simulink model "ASSIGN_pe_q12"  (R2025b)
settings: Solver=VariableStepAuto  StartTime=0.0  StopTime=0.5  RelTol=1e-3
libraries: spsACVoltageSourceLib x3, spsThyristorLib x3, spsGroundLib x2, spsRMSLib x2, spsVoltageMeasurementLib x2, spsCurrentMeasurementLib x1, spsMeanLib x1, spsPower3phInstantaneousLib x1, spsSeriesRLCBranchLib x1, spsThreePhaseVIMeasurementLib x1, sps_lib x1
settings Model: Creator=Luqmaan  LastModifiedBy=Luqmaan

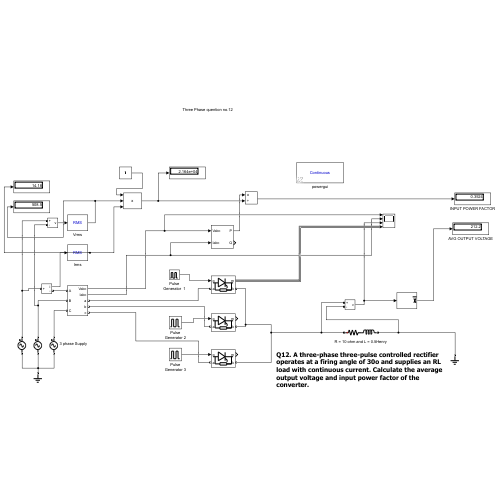
[thumbnail: Simulink's stored preview of the top-level diagram]
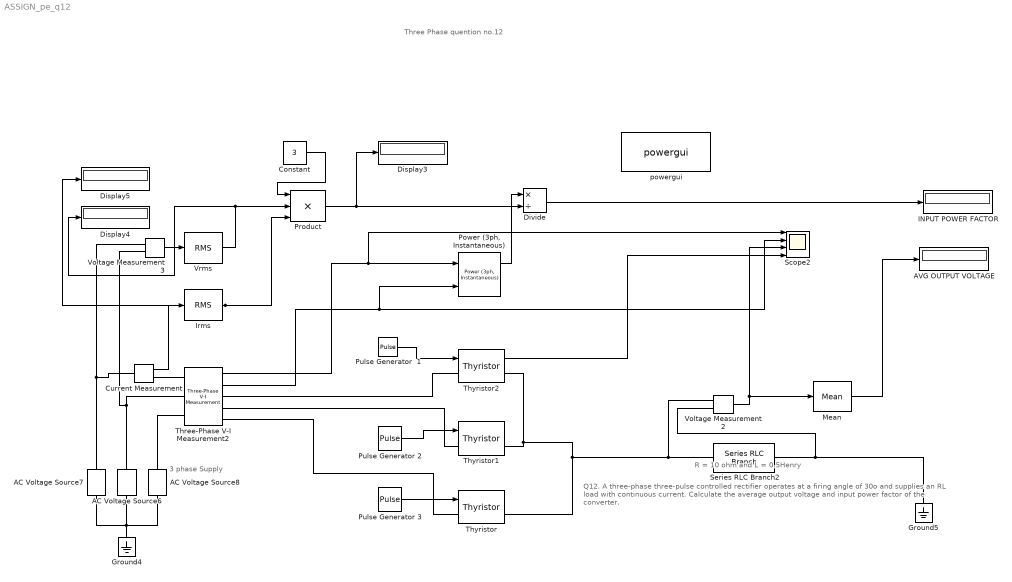
== system ASSIGN_pe_q12 ==
  note: Q12. A three-phase three-pulse controlled rectifier operates at a firing angle of 30o and supplies an RL load with continuous current. Calculate the average output voltage and input power factor of the converter.
  note: 3 phase Supply
  note: R = 10 ohm and L = 0.5Henry
  note: Three Phase quention no.12
  AC Voltage Source6 : spsACVoltageSourceLib/AC Voltage Source  Amplitude=415  Phase=120  Frequency=50  SampleTime=0  Measurements=None  BusType=swing  Pref=10e3  Qref=0  Qmin=-inf  Qmax=+inf
  AC Voltage Source7 : spsACVoltageSourceLib/AC Voltage Source  Amplitude=415  Phase=0  Frequency=50  SampleTime=0  Measurements=None  BusType=swing  Pref=10e3  Qref=0  Qmin=-inf  Qmax=+inf
  AC Voltage Source8 : spsACVoltageSourceLib/AC Voltage Source  Amplitude=415  Phase=240  Frequency=50  SampleTime=0  Measurements=None  BusType=swing  Pref=10e3  Qref=0  Qmin=-inf  Qmax=+inf
  AVG OUTPUT VOLTAGE : Display
  Constant : Constant  Value=3
  Current Measurement : spsCurrentMeasurementLib/Current Measurement  PhasorSimulation=off  OutputType=Complex  PSBequivalent=0
  Display3 : Display
  Display4 : Display
  Display5 : Display
  Divide : Product  Inputs=*/
  Ground4 : spsGroundLib/Ground  LConnTagsString=a
  Ground5 : spsGroundLib/Ground  LConnTagsString=a
  INPUT POWER FACTOR : Display
  Irms : spsRMSLib/RMS  TrueRMS=on  Freq=50  RMSInit=120  Ts=0
  Mean : spsMeanLib/Mean  Freq=50  Vinit=0  Ts=0
  "Power (3ph, Instantaneous)" : spsPower3phInstantaneousLib/Power (3ph, Instantaneous)
  Product : Product  Inputs=3
  Pulse Generator  1 : DiscretePulseGenerator  PulseType=Time based  Period=0.02  PulseWidth=10  PhaseDelay=60*(0.02/360)
  Pulse Generator 2 : DiscretePulseGenerator  PulseType=Time based  Period=0.02  PulseWidth=10  PhaseDelay=210*(0.02/360)
  Pulse Generator 3 : DiscretePulseGenerator  PulseType=Time based  Period=0.02  PulseWidth=10  PhaseDelay=300*(0.02/360)
  Scope2 : Scope  NumInputPorts=4
      settings: ActiveDisplayYMinimum=-499.99999999591512  ActiveDisplayYMaximum=499.99999999954611  DataLoggingVariableName=ScopeData2
  Series RLC Branch2 : spsSeriesRLCBranchLib/Series RLC Branch  LConnTagsString=__new0  RConnTagsString=__new0  BranchType=RL  Resistance=10  Inductance=0.5  SetiL0=off  InitialCurrent=0  Capacitance=1e-6  Setx0=off  InitialVoltage=0  Measurements=None
  Three-Phase V-I Measurement2 : spsThreePhaseVIMeasurementLib/Three-Phase V-I Measurement  VoltageMeasurement=phase-to-ground  SetLabelV=off  LabelV=Vabc  Vpu=off  VpuLL=off  CurrentMeasurement=yes  SetLabelI=off  LabelI=Iabc  Ipu=off  Pbase=100e6  Vbase=500e3  OutputType=Complex  PhasorSimulation=off  PSBequivalent=0
  Thyristor : spsThyristorLib/Thyristor  Ron=0.001  Lon=0  Vf=0.8  IC=0  Rs=500  Cs=250e-9  Measurements=on
  Thyristor1 : spsThyristorLib/Thyristor  Ron=0.001  Lon=0  Vf=0.8  IC=0  Rs=500  Cs=250e-9  Measurements=on
  Thyristor2 : spsThyristorLib/Thyristor  Ron=0.001  Lon=0  Vf=0.8  IC=0  Rs=500  Cs=250e-9  Measurements=on
  Voltage Measurement2 : spsVoltageMeasurementLib/Voltage Measurement  PhasorSimulation=off  OutputType=Complex  PSBequivalent=0
  Voltage Measurement3 : spsVoltageMeasurementLib/Voltage Measurement  PhasorSimulation=off  OutputType=Complex  PSBequivalent=0
  Vrms : spsRMSLib/RMS  TrueRMS=on  Freq=50  RMSInit=120  Ts=0
  powergui : sps_lib/powergui  Priority=1  SimulationMode=Continuous  SampleTime=50e-6  frequency=60  Iterations=50  frequencyindice=50  Pbase=100e6  ErrMax=1e-4  UnitsV=kV  UnitsW=MW  buscounter=0  FunctionMessages=off  echomessages=off  EnableUseOfTLC=off  CurrentSourceSwitches=off  DisableSnubberDevices=off  DisableRonSwitches=off  DisableVfSwitches=off  DisplayEquations=off  AutomaticDiscreteSolvers=off  SolverType=Tustin/Backward Euler (TBE)  Interpol=off  ExternalGateDelay=off  methode=off  Ts=100  x0status=blocks  SPID=on  SwTol=0  HookPort=off  NonlinearTolerance=1e-4  nMaxIteration=100  ContinueOnMaxIteration=off  RestoreLinks=warning  ResistiveCurrentMeasurement=off  Frange=[0:2:500]  Ylog=off  Xlog=on  ShowGrid=off  save=off  variable=ZData  structure=0  ZoomFFT=off  StartTime=0.0  cycles=1  DisplayStyle=1  fundamental=60  FreqAxis=off  MaxFrequency=1000  frequencyindicesteady=1  RmsSteady=1  display=off
  wires:
  Three-Phase V-I Measurement2/2 -> "Power (3ph, Instantaneous)"/2, Scope2/2
  Pulse Generator 2/1 -> Thyristor1/1
  Three-Phase V-I Measurement2/1 -> Scope2/1, "Power (3ph, Instantaneous)"/1
  Pulse Generator 3/1 -> Thyristor/1
  Pulse Generator  1/1 -> Thyristor2/1
  Mean/1 -> AVG OUTPUT VOLTAGE/1
  Voltage Measurement2/1 -> Scope2/3, Mean/1
  Thyristor2/1 -> Scope2/4
  Voltage Measurement3/1 -> Vrms/1
  Current Measurement/1 -> Irms/1
  Constant/1 -> Product/1
  Vrms/1 -> Product/2, Display4/1
  Irms/1 -> Product/3, Display5/1
  "Power (3ph, Instantaneous)"/1 -> Divide/1
  Product/1 -> Display3/1, Divide/2
  Divide/1 -> INPUT POWER FACTOR/1
  connections:
  AC Voltage Source7/LConn1 -- Ground4/LConn1 -- AC Voltage Source6/LConn1 -- AC Voltage Source8/LConn1
  Voltage Measurement2/LConn2 -- Series RLC Branch2/RConn1 -- Ground5/LConn1
  Voltage Measurement2/LConn1 -- Series RLC Branch2/LConn1 -- Thyristor/RConn1 -- Thyristor1/RConn1 -- Thyristor2/RConn1
  Three-Phase V-I Measurement2/RConn3 -- Thyristor/LConn1
  AC Voltage Source6/RConn1 -- Three-Phase V-I Measurement2/LConn2 -- Voltage Measurement3/LConn2
  Three-Phase V-I Measurement2/RConn2 -- Thyristor1/LConn1
  Three-Phase V-I Measurement2/RConn1 -- Thyristor2/LConn1
  AC Voltage Source8/RConn1 -- Three-Phase V-I Measurement2/LConn3
  AC Voltage Source7/RConn1 -- Voltage Measurement3/LConn1 -- Current Measurement/LConn1
  Current Measurement/RConn1 -- Three-Phase V-I Measurement2/LConn1
